simulink model "open_loop"  (R2021b)
settings: Solver=VariableStepAuto  StartTime=0.0  StopTime=100.0  RelTol=1e-3
values from neighbouring files (symbols this model uses):
  A = zeros(size(B'))    [parameters.m]
  I = 4000*eye(3)    [parameters.m]
  Iz = I(end)    [particle_mpc.m]
  m = length(arch_type)    [batch_simulation.m]    (also in particle_mpc.m = mass)
  mass = 2000    [parameters.m]
  r_1 = [front_length;width/2;-height]    [parameters.m]
  radius = 0.4    [parameters.m]
  rear_length = 1.6    [parameters.m]
  sys_d = c2d(sys, ts)    [particle_mpc.m]
  ts = 0.5    [particle_mpc.m]
libraries: nesl_utility x9, autolibshared x5, vrlib x4, mpclib x1
(part 1 of 4)
settings Model: Creator=Zephyrus  LastModifiedBy=Zephyrus

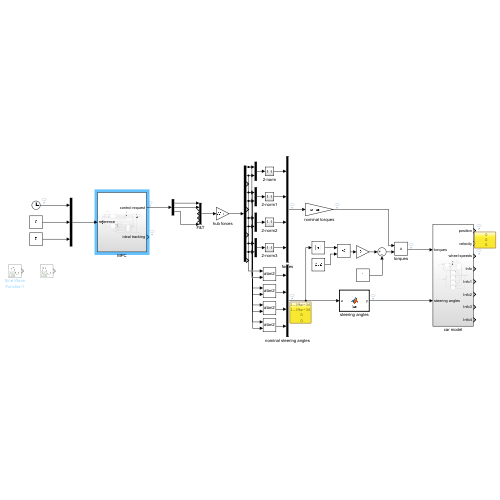
[thumbnail: Simulink's stored preview of the top-level diagram]
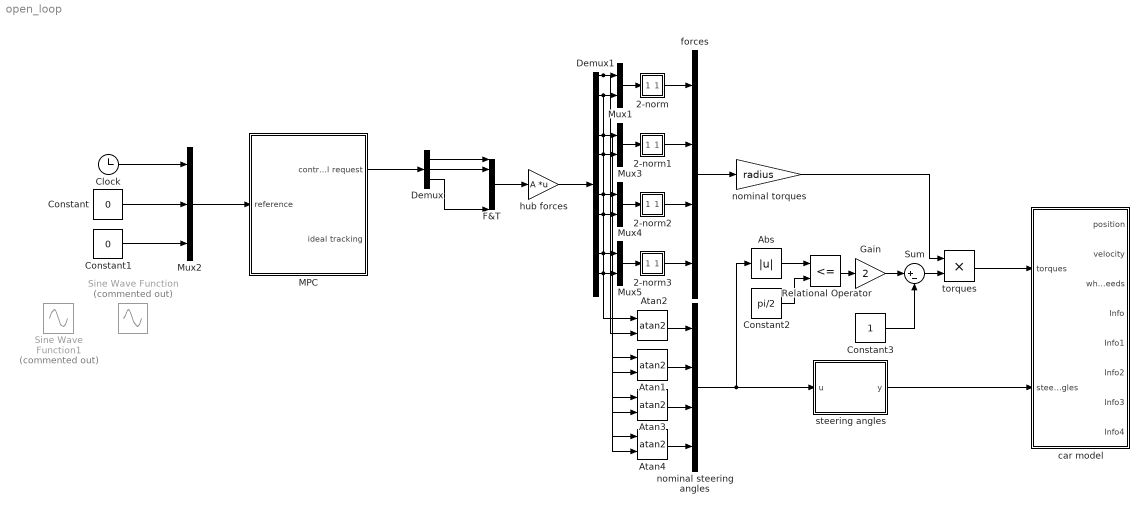
== system open_loop ==
  2-norm : Subsystem
  2-norm1 : Subsystem
  2-norm2 : Subsystem
  2-norm3 : Subsystem
  Abs : Abs
  Atan{1..4} (4 alike) : Trigonometry  Operator=atan2
  Clock : Clock
  Constant : Constant  Value=0
  Constant1 : Constant  Value=0
  Constant2 : Constant  Value=pi/2
  Constant3 : Constant
  Demux : Demux  Outputs=3
  Demux1 : Demux  Outputs=12
  F&T : Mux  Inputs=6
  Gain : Gain  Gain=2
  MPC : Subsystem
  Mux{1,3..5} (4 alike) : Mux  Inputs=2
  Mux2 : Mux  Inputs=3
  Relational Operator : RelationalOperator  Operator=<=  OutDataTypeStr=boolean  RndMeth=Simplest
  Sine Wave Function : Sin  Commented=on  SampleTime=0
  Sine Wave Function1 : Sin  Commented=on  Phase=pi/2  SampleTime=0
  Sum : Sum  Inputs=|+-
  car model : Subsystem
  forces : Mux
  hub forces : Gain  Gain=A  Multiplication=Matrix(K*u)
  nominal steering angles : Mux
  nominal torques : Gain  Gain=radius
  steering angles : MATLAB Function  TreatAsAtomicUnit=on
  torques : Product
  wires:
  Clock/1 -> Mux2/1
  Mux2/1 -> MPC/1(reference)
  MPC/1(control request) -> Demux/1
  Demux/2 -> F&T/2
  Demux/1 -> F&T/1
  Demux/3 -> F&T/6
  F&T/1 -> hub forces/1
  Demux1/1 -> Atan2/2, Mux1/1
  Demux1/2 -> Atan2/1, Mux1/2
  hub forces/1 -> Demux1/1
  Demux1/4 -> Atan1/2, Mux3/1
  Demux1/5 -> Atan1/1, Mux3/2
  Demux1/7 -> Atan3/2, Mux4/1
  Demux1/8 -> Atan3/1, Mux4/2
  Demux1/10 -> Atan4/2, Mux5/1
  Demux1/11 -> Atan4/1, Mux5/2
  Mux1/1 -> 2-norm/1(In1)
  Mux3/1 -> 2-norm1/1(In1)
  Mux5/1 -> 2-norm3/1(In1)
  Mux4/1 -> 2-norm2/1(In1)
  2-norm/1(Out1) -> forces/1
  2-norm1/1(Out1) -> forces/2
  2-norm2/1(Out1) -> forces/3
  2-norm3/1(Out1) -> forces/4
  Atan2/1 -> nominal steering angles/1
  Atan1/1 -> nominal steering angles/2
  Atan3/1 -> nominal steering angles/3
  Atan4/1 -> nominal steering angles/4
  forces/1 -> nominal torques/1
  Constant/1 -> Mux2/2
  Constant1/1 -> Mux2/3
  Abs/1 -> Relational Operator/1
  nominal steering angles/1 -> Abs/1, steering angles/1(u)
  Constant2/1 -> Relational Operator/2
  steering angles/1(y) -> car model/2(steering angles)
  Relational Operator/1 -> Gain/1
  nominal torques/1 -> torques/1
  torques/1 -> car model/1(torques)
  Gain/1 -> Sum/1
  Sum/1 -> torques/2
  Constant3/1 -> Sum/2

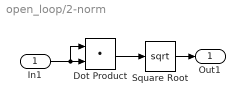
== system open_loop/2-norm ==
  In1 : Inport
  Dot Product : DotProduct  InputSameDT=on  OutDataTypeStr=Inherit: Inherit via internal rule
  Square Root : Sqrt  SaturateOnIntegerOverflow=on
  Out1 : Outport
  wires:
  Square Root/1 -> Out1/1
  Dot Product/1 -> Square Root/1
  In1/1 -> Dot Product/1, Dot Product/2

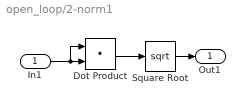
== system open_loop/2-norm1 ==
  In1 : Inport
  Dot Product : DotProduct  InputSameDT=on  OutDataTypeStr=Inherit: Inherit via internal rule
  Square Root : Sqrt  SaturateOnIntegerOverflow=on
  Out1 : Outport
  wires:
  Square Root/1 -> Out1/1
  Dot Product/1 -> Square Root/1
  In1/1 -> Dot Product/1, Dot Product/2

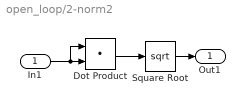
== system open_loop/2-norm2 ==
  In1 : Inport
  Dot Product : DotProduct  InputSameDT=on  OutDataTypeStr=Inherit: Inherit via internal rule
  Square Root : Sqrt  SaturateOnIntegerOverflow=on
  Out1 : Outport
  wires:
  Square Root/1 -> Out1/1
  Dot Product/1 -> Square Root/1
  In1/1 -> Dot Product/1, Dot Product/2

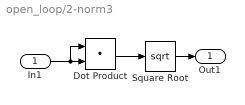
== system open_loop/2-norm3 ==
  In1 : Inport
  Dot Product : DotProduct  InputSameDT=on  OutDataTypeStr=Inherit: Inherit via internal rule
  Square Root : Sqrt  SaturateOnIntegerOverflow=on
  Out1 : Outport
  wires:
  Square Root/1 -> Out1/1
  Dot Product/1 -> Square Root/1
  In1/1 -> Dot Product/1, Dot Product/2

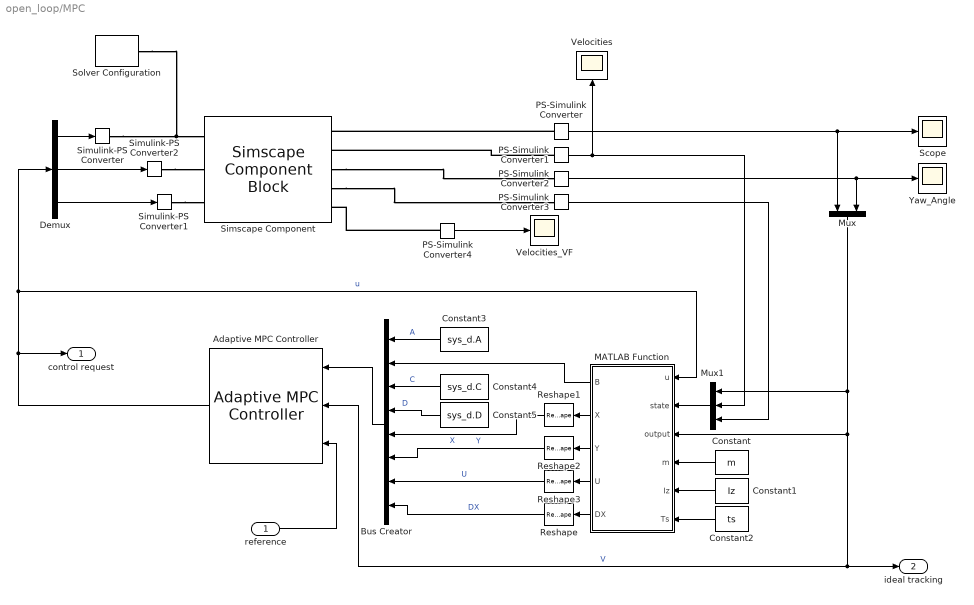
== system open_loop/MPC ==
  reference : Inport
  Adaptive MPC Controller : mpclib/Adaptive MPC Controller  SCDEnableBlockLinearizationSpecification=on  mpcobj=mpc_controller  enable_value=0  updateMPCinCallerWorkspace=on  md_inport=off  mv_inport=off  uref_inport=off  return_cost=off  return_mvseq=off  return_qpstatus=off  return_xseq=off  return_state=off  return_ovseq=off  state_inport=off  isltv_plant=off  umin_inport=off  umax_inport=off  ymin_inport=off  ymax_inport=off  cc_inport=off  ywt_inport=off  uwt_inport=off  duwt_inport=off  rhoeps_inport=off  pm_inport=off  MaximumP=10  HorizonChoice=FixedHorizon  BlockDataType=double  SampleTimeInherited=off  switch_inport=off
  Bus Creator : BusCreator  Inputs=8
  Constant : Constant  Value=m
  Constant1 : Constant  Value=Iz
  Constant2 : Constant  Value=ts
  Constant3 : Constant  Value=sys_d.A
  Constant4 : Constant  Value=sys_d.C
  Constant5 : Constant  Value=sys_d.D
  Demux : Demux  Outputs=3
  MATLAB Function : MATLAB Function  TreatAsAtomicUnit=on
  Mux : Mux  Inputs=2
  Mux1 : Mux  Inputs=3
  PS-Simulink Converter{,1..4} (5 alike) : nesl_utility/PS-Simulink Converter  PhysicalDomain=network_engine_domain  SubClassName=ps_output  LeftPortType=input  RightPortType=output  PseudoPeriodic=off  Frequencies=[]  Unit=inherit  AffineConversion=off
      settings: SourceProductBaseCode=PW,SS
  Reshape : Reshape  OutputDimensionality=Customize  OutputDimensions=[6, 1]
  Reshape1 : Reshape  OutputDimensionality=Customize  OutputDimensions=[6, 1]
  Reshape2 : Reshape  OutputDimensionality=Customize  OutputDimensions=[3, 1]
  Reshape3 : Reshape  OutputDimensionality=Customize  OutputDimensions=[3, 1]
  Scope : Scope
  Simscape Component : SimscapeComponentBlock  SourceFile=particle  ComponentPath=particle  ComponentVariants="[\"particle\"]"  ComponentVariantNames="[\"particle\"]"  ClassName=particle  SchemaVersion=1  mass=mass kg  Iz=I(end) kg*m^2  x_specify=off  x_priority=None  x=0 m  x_nominal_specify=off  x_nominal_unit=m  x_nominal_value=1  dx_specify=off  dx_priority=None  dx=0 m/s  dx_nominal_specify=off  dx_nominal_unit=m/s  dx_nominal_value=1  y_specify=off  y_priority=None  y=0 m  y_nominal_specify=off  y_nominal_unit=m  y_nominal_value=1  dy_specify=off  dy_priority=None  dy=0 m/s  dy_nominal_specify=off  dy_nominal_unit=m/s  dy_nominal_value=1  theta_specify=on  theta_priority=None  theta=0 rad  theta_nominal_specify=off  theta_nominal_unit=rad  theta_nominal_value=1  dtheta_specify=off  dtheta_priority=None  dtheta=0 rad/s  dtheta_nominal_specify=off  dtheta_nominal_unit=rad/s  dtheta_nominal_value=1
      settings: CopyFcn=simscape.engine.sli.internal.componentblockcallback(gcbh,'COPY')  PreCopyFcn=simscape.engine.sli.internal.componentblockcallback(gcbh,'PRECOPY')  PreDeleteFcn=simscape.engine.sli.internal.componentblockcallback(gcbh,'PREDELETE')  InternalSimscapePortConfiguration="{\"Bottom\":[],\"Left\":[{\"id\":\"fx\",\"label\":\"fx\",\"type\":\"input\"},{\"id\":\"fy\",\"label\":\"fy\",\"type\":\"input\"},{\"id\":\"Mz\",\"label\":\"Mz\",\"type\":\"input\"}],\"Right\":[{\"id\":\"pos\",\"label\":\"pos\",\"type\":\"output\"},{\"id\":\"velocity\",\"label\":\"velocity\",\"type\":\"output\"},{\"id\":\"angle\",\"label\":\"angle\",\"type\":\"output\"},{\"id\":\"angular_vel\",\"label\":\"angular_vel\",\"type\":\"output\"},{\"id\":\"velocity_VF\",\"label\":\"velocity_VF\",\"type\":\"output\"}],\"Top\":[]}"
      mask Type: particle
  Simulink-PS Converter : nesl_utility/Simulink-PS Converter  PhysicalDomain=network_engine_domain  SubClassName=ps_input  LeftPortType=input  RightPortType=output  PseudoPeriodic=off  Frequencies=[]  NoiseDistribution=none  NoiseParameters=[]  Unit=1  AffineConversion=off  FilteringAndDerivatives=provide  SimscapeFilterOrder=1  InputFilterTimeConstant=0.001  UdotUserProvided=0
      settings: SourceProductBaseCode=PW,SS
  Simulink-PS Converter1 : nesl_utility/Simulink-PS Converter  PhysicalDomain=network_engine_domain  SubClassName=ps_input  LeftPortType=input  RightPortType=output  PseudoPeriodic=off  Frequencies=[]  NoiseDistribution=none  NoiseParameters=[]  Unit=1  AffineConversion=off  FilteringAndDerivatives=provide  SimscapeFilterOrder=1  InputFilterTimeConstant=0.001  UdotUserProvided=0
      settings: SourceProductBaseCode=PW,SS
  Simulink-PS Converter2 : nesl_utility/Simulink-PS Converter  PhysicalDomain=network_engine_domain  SubClassName=ps_input  LeftPortType=input  RightPortType=output  PseudoPeriodic=off  Frequencies=[]  NoiseDistribution=none  NoiseParameters=[]  Unit=1  AffineConversion=off  FilteringAndDerivatives=provide  SimscapeFilterOrder=1  InputFilterTimeConstant=0.001  UdotUserProvided=0
      settings: SourceProductBaseCode=PW,SS
  Solver Configuration : nesl_utility/Solver Configuration  PhysicalDomain=network_engine_domain  SubClassName=solver  LeftPortType=input  RightPortType=generic  Tones=[]  Harmonics=[]  SimulateNoise=off  Profile=off  UseLocalSampling=off  EnableSwitchedLinearOptims=on  FrequencyDomain=off  UseCCode=off  RelTol=0.001  AbsTol=1e-06  MinStep=1e-09  ToWorkspace=off  RevertToSquareIcSolve=off  NumHomotopyIterations=100  PhasorMode=off  PhasorModeNumHarmonics=1  DoDC=off  ResidualTolerance=1e-09  UseLocalSolver=off  LocalSolverChoice=NE_BACKWARD_EULER_ADVANCER  LocalSolverSampleTime=0.001  DoFixedCost=off  MaxNonlinIter=3  MaxModeIter=2  ComputeImpulses=off  ImpulseIterations=2  LinearAlgebra=auto  EquationFormulation=NE_TIME_EF  DelaysMemoryBudget=1024  AutomaticFiltering=on  FilteringTimeConstant=0.001  PartitionStorageMethod=AS_NEEDED  PartitionMemoryBudget=1024  PartitionMethod=ROBUST
      settings: SourceProductBaseCode=PW,SS
  Velocities : Scope
  Velocities_VF : Scope
  Yaw_Angle : Scope
  control request : Outport
  ideal tracking : Outport  Port=2
  wires:
  Demux/3 -> Simulink-PS Converter1/1
  MATLAB Function/3(Y) -> Reshape2/1
  Constant/1 -> MATLAB Function/4(m)
  MATLAB Function/5(DX) -> Reshape/1
  MATLAB Function/1(B) -> Bus Creator/2
  Adaptive MPC Controller/1 -> control request/1, MATLAB Function/1(u), Demux/1  "u"
  MATLAB Function/4(U) -> Reshape3/1
  Mux1/1 -> MATLAB Function/2(state)
  Mux/1 -> Mux1/1, MATLAB Function/3(output), Adaptive MPC Controller/2, ideal tracking/1  "V"
  PS-Simulink Converter2/1 -> Mux/2, Yaw_Angle/1
  Constant2/1 -> MATLAB Function/6(Ts)
  Constant5/1 -> Bus Creator/4  "D"
  Reshape3/1 -> Bus Creator/7  "U"
  Constant3/1 -> Bus Creator/1  "A"
  PS-Simulink Converter3/1 -> Mux1/3
  Reshape2/1 -> Bus Creator/6  "Y"
  Demux/2 -> Simulink-PS Converter2/1
  Constant1/1 -> MATLAB Function/5(Iz)
  Reshape/1 -> Bus Creator/8  "DX"
  PS-Simulink Converter1/1 -> Mux1/2, Velocities/1
  Demux/1 -> Simulink-PS Converter/1
  PS-Simulink Converter/1 -> Mux/1, Scope/1
  Reshape1/1 -> Bus Creator/5  "X"
  PS-Simulink Converter4/1 -> Velocities_VF/1
  Bus Creator/1 -> Adaptive MPC Controller/1
  MATLAB Function/2(X) -> Reshape1/1
  Constant4/1 -> Bus Creator/3  "C"
  reference/1 -> Adaptive MPC Controller/3
  connections:
  PS-Simulink Converter4/LConn1 -- Simscape Component/RConn5
  Simulink-PS Converter2/RConn1 -- Simscape Component/LConn2
  Solver Configuration/RConn1 -- Simulink-PS Converter/RConn1 -- Simscape Component/LConn1
  PS-Simulink Converter1/LConn1 -- Simscape Component/RConn2
  Simulink-PS Converter1/RConn1 -- Simscape Component/LConn3
  PS-Simulink Converter/LConn1 -- Simscape Component/RConn1
  Simscape Component/RConn4 -- PS-Simulink Converter3/LConn1
  Simscape Component/RConn3 -- PS-Simulink Converter2/LConn1
